simulink model "continuization_model"  (R2018b)
settings: Solver=FixedStepAuto  StartTime=0.0  StopTime=5  FixedStep=1e-4  RelTol=1e-3
values from neighbouring files (symbols this model uses):
  A = 0    [example_f1_f2.m]
  B = 3    [example_f1_f2.m]
  K = -1    [example_f1_f2.m]
  L = 0    [example_f1_f2.m]
  omega_dot = 0    [example_f1_f2.m]
  T = 1    [example_f1_f2.m]
  x_c_0_cont = K * x_p_0 + L * x_c_0    (= -1)    [example_f1_f2.m]
  x_p_0 = 1    [example_f1_f2.m]
libraries: dspsigops x1
settings Model: Creator=ak22emur  LastModifiedBy=ak22emur

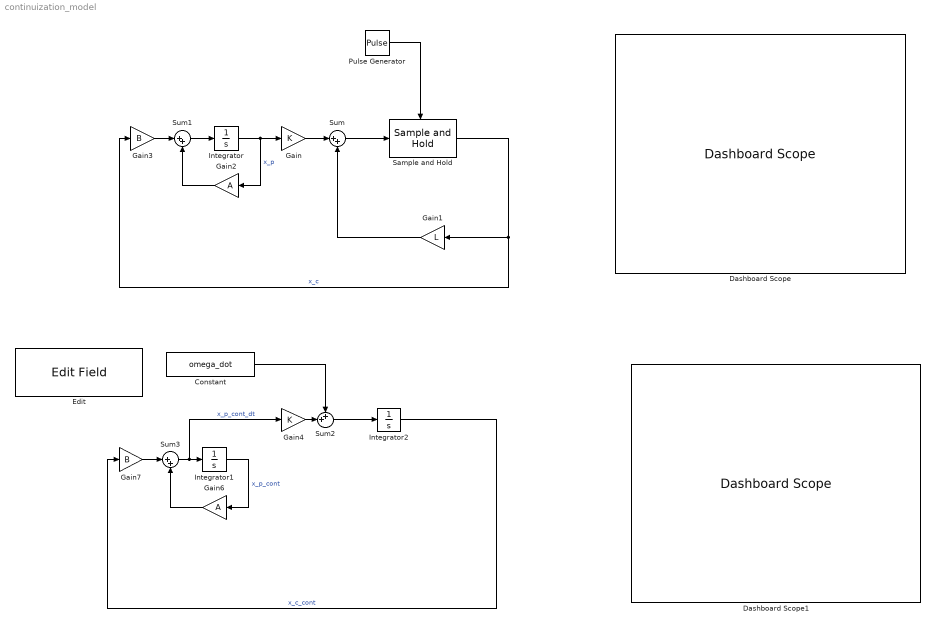
== system continuization_model ==
  Constant : Constant  Value=omega_dot
  Dashboard Scope : DashboardScope  WebBlockId=26
  Dashboard Scope1 : DashboardScope  WebBlockId=27
  Edit : EditField  WebBlockId=28  ShowInitialText=on  Alignment=Center
  Gain : Gain  Gain=K
  Gain1 : Gain  Gain=L
  Gain2 : Gain  Gain=A
  Gain3 : Gain  Gain=B
  Gain4 : Gain  Gain=K
  Gain6 : Gain  Gain=A
  Gain7 : Gain  Gain=B
  Integrator : Integrator  InitialCondition=x_p_0
  Integrator1 : Integrator  InitialCondition=x_p_0
  Integrator2 : Integrator  InitialCondition=x_c_0_cont
  Pulse Generator : DiscretePulseGenerator  PulseType=Time based  Period=T  PulseWidth=5
  Sample and Hold : dspsigops/Sample and Hold  trig=Rising edge  initCond=x_c_0  latchinput=on
  Sum : Sum  Inputs=|++
  Sum1 : Sum  Inputs=|++
  Sum2 : Sum  Inputs=++|
  Sum3 : Sum  Inputs=|++
  wires:
  Sample and Hold/1 -> Gain3/1, Gain1/1  "x_c"
  Pulse Generator/1 -> Sample and Hold/Trigger
  Sum/1 -> Sample and Hold/1
  Gain/1 -> Sum/1
  Gain1/1 -> Sum/2
  Integrator/1 -> Gain2/1, Gain/1  "x_p"
  Sum1/1 -> Integrator/1
  Gain2/1 -> Sum1/2
  Gain3/1 -> Sum1/1
  Gain7/1 -> Sum3/1
  Integrator2/1 -> Gain7/1  "x_c_cont"
  Sum2/1 -> Integrator2/1
  Sum3/1 -> Gain4/1, Integrator1/1  "x_p_cont_dt"
  Integrator1/1 -> Gain6/1  "x_p_cont"
  Gain6/1 -> Sum3/2
  Gain4/1 -> Sum2/2
  Constant/1 -> Sum2/1
